simulink model "EHB_MOTOR"  (R2023b)
settings: Solver=FixedStepDiscrete  StartTime=0.0  StopTime=inf  FixedStep=0.0001  RelTol=1e-3  EnableMultiTasking=on
undefined symbols (not defined in the file): CAN_EHB_VCU0x125, CAN_EHB_VCU0x126, CAN_id0x120_Data, Cos_Table, Cos_Table1, EHB_DTC_status, R, Sin_BreakPoint, Sin_BreakPoint1, Sin_Table, Sin_Table1, T
libraries: simulink x30
(part 6 of 9)

== system EHB_MOTOR/EPB_CTRL/EPB_Diag/EPBOverheatDiag/Subsystem1 ==
  note: 控制器温度超过限定值
  In1 : Inport
  function : TriggerPort  TriggerType=function-call  VariantControl=Variant
  Constant : Constant  Value=0  OutDataTypeStr=uint8
  Data Store Memory1 : DataStoreMemory  DataStoreName=EPBTempOverride_C  ReadBeforeWriteMsg=warning  WriteAfterWriteMsg=warning  WriteAfterReadMsg=warning  ShowAdditionalParam=off  OutDataTypeStr=uint16
  Data Store Memory5 : DataStoreMemory  DataStoreName=EPBTempMAX_C  ReadBeforeWriteMsg=warning  WriteAfterWriteMsg=warning  WriteAfterReadMsg=warning  ShowAdditionalParam=off  OutDataTypeStr=uint16
  Data Store Read : DataStoreRead  DataStoreName=EPBTempOverride_C  DataStoreElements=EPBTempOverride_C  IndexOptions=Index vector (dialog)  Indices=1  OutputSizes=1
  Data Store Read2 : DataStoreRead  DataStoreName=EPBTempMAX_C  DataStoreElements=EPBTempMAX_C  IndexOptions=Index vector (dialog)  Indices=1  OutputSizes=1
  ErrorSignalCount : Stateflow chart  TreatAsAtomicUnit=on
  Relational Operator1 : RelationalOperator  Operator=>  OutDataTypeStr=boolean  RndMeth=Simplest  InputSameDT=off
  Out1 : Outport  VectorParamsAs1DForOutWhenUnconnected=off
  wires:
  ErrorSignalCount/1(EPBTempOverride) -> Out1/1
  Relational Operator1/1 -> ErrorSignalCount/1(EPBTemp)
  Data Store Read/1 -> ErrorSignalCount/2(EPBTempOverride_C)
  Constant/1 -> ErrorSignalCount/3(Recover)
  In1/1 -> Relational Operator1/1
  Data Store Read2/1 -> Relational Operator1/2

== system EHB_MOTOR/EPB_CTRL/EPB_Diag/EPB_vBATDiag/Subsystem ==
  note: 电源电压过低
  note: 16V
  note: 10V
  note: 电源电压过高
  In1 : Inport
  function : TriggerPort  TriggerType=function-call  VariantControl=Variant
  Constant : Constant  Value=0  OutDataTypeStr=uint8
  Constant1 : Constant  Value=0  OutDataTypeStr=uint8
  Data Store Memory1 : DataStoreMemory  DataStoreName=EPBVoltage_C  ReadBeforeWriteMsg=warning  WriteAfterWriteMsg=warning  WriteAfterReadMsg=warning  ShowAdditionalParam=off  OutDataTypeStr=uint16
  Data Store Memory4 : DataStoreMemory  DataStoreName=EPBVoltageMIN_C  ReadBeforeWriteMsg=warning  WriteAfterWriteMsg=warning  WriteAfterReadMsg=warning  ShowAdditionalParam=off  OutDataTypeStr=uint16
  Data Store Memory5 : DataStoreMemory  DataStoreName=EPBVoltageMAX_C  ReadBeforeWriteMsg=warning  WriteAfterWriteMsg=warning  WriteAfterReadMsg=warning  ShowAdditionalParam=off  OutDataTypeStr=uint16
  Data Store Read : DataStoreRead  DataStoreName=EPBVoltage_C  DataStoreElements=EPBVoltage_C  IndexOptions=Index vector (dialog)  Indices=1  OutputSizes=1
  Data Store Read1 : DataStoreRead  DataStoreName=EPBVoltageMIN_C  DataStoreElements=EPBVoltageMIN_C  IndexOptions=Index vector (dialog)  Indices=1  OutputSizes=1
  Data Store Read2 : DataStoreRead  DataStoreName=EPBVoltageMAX_C  DataStoreElements=EPBVoltageMAX_C  IndexOptions=Index vector (dialog)  Indices=1  OutputSizes=1
  Data Store Read3 : DataStoreRead  DataStoreName=EPBVoltage_C  DataStoreElements=EPBVoltage_C  IndexOptions=Index vector (dialog)  Indices=1  OutputSizes=1
  ErrorSignalCount : Stateflow chart  TreatAsAtomicUnit=on
  ErrorSignalCount1 : Stateflow chart  TreatAsAtomicUnit=on
  Relational Operator : RelationalOperator  Operator=<  OutDataTypeStr=boolean  RndMeth=Simplest  InputSameDT=off
  Relational Operator1 : RelationalOperator  Operator=>  OutDataTypeStr=boolean  RndMeth=Simplest  InputSameDT=off
  Out1 : Outport  VectorParamsAs1DForOutWhenUnconnected=off
  Out2 : Outport  Port=2  VectorParamsAs1DForOutWhenUnconnected=off
  wires:
  ErrorSignalCount/1(EPBVoltageMAX) -> Out2/1
  Relational Operator1/1 -> ErrorSignalCount/1(EPBVoltage)
  Data Store Read3/1 -> ErrorSignalCount/2(EPBVoltageMAX_C)
  Constant1/1 -> ErrorSignalCount/3(Recover)
  Constant/1 -> ErrorSignalCount1/3(Recover)
  Data Store Read/1 -> ErrorSignalCount1/2(EPBVoltageMIN_C)
  Relational Operator/1 -> ErrorSignalCount1/1(EPBVoltage)
  ErrorSignalCount1/1(EPBVoltageMIN) -> Out1/1
  Data Store Read2/1 -> Relational Operator1/2
  In1/1 -> Relational Operator/1, Relational Operator1/1
  Data Store Read1/1 -> Relational Operator/2

== system EHB_MOTOR/EPB_CTRL/Subsystem1/EPB_interface/12vADC2VOLT ==
  EPB_vBAT_AD : Inport
  Filter : Subsystem  Commented=on
  vMCU2PIN : Subsystem
  EPB_vBAT_filtered : Outport  VectorParamsAs1DForOutWhenUnconnected=off
  wires:
  EPB_vBAT_AD/1 -> vMCU2PIN/1(EPB_vBAT_AD)
  vMCU2PIN/1(EPB_vBAT) -> EPB_vBAT_filtered/1

== system EHB_MOTOR/EPB_CTRL/Subsystem1/EPB_interface/EPB1DC2Cur ==
  EPB1_Current_AD : Inport
  Data Store Memory : DataStoreMemory  DataStoreName=EPB1_actCurent  ReadBeforeWriteMsg=warning  WriteAfterWriteMsg=warning  WriteAfterReadMsg=warning  ShowAdditionalParam=off  OutDataTypeStr=double
  Data Store Write : DataStoreWrite  DataStoreName=EPB1_actCurent  DataStoreElements=EPB1_actCurent  IndexOptions=Index vector (dialog)  Indices=1  OutputSizes=1
  Filter : Subsystem  Commented=on
  vMCU2PIN : Subsystem
  EPB1_Current_filtered : Outport  VectorParamsAs1DForOutWhenUnconnected=off
  wires:
  EPB1_Current_AD/1 -> vMCU2PIN/1(EPB1_Current_AD)
  vMCU2PIN/1(EPB1_Current) -> Data Store Write/1, EPB1_Current_filtered/1

== system EHB_MOTOR/EPB_CTRL/Subsystem1/EPB_interface/EPB2DC2Cur ==
  EPB2_Current_AD : Inport
  Data Store Memory : DataStoreMemory  DataStoreName=EPB2_actCurent  ReadBeforeWriteMsg=warning  WriteAfterWriteMsg=warning  WriteAfterReadMsg=warning  ShowAdditionalParam=off  OutDataTypeStr=double
  Data Store Write : DataStoreWrite  DataStoreName=EPB2_actCurent  DataStoreElements=EPB2_actCurent  IndexOptions=Index vector (dialog)  Indices=1  OutputSizes=1
  Filter : Subsystem  Commented=on
  vMCU2PIN : Subsystem
  EPB2_Current_filtered : Outport  VectorParamsAs1DForOutWhenUnconnected=off
  wires:
  EPB2_Current_AD/1 -> vMCU2PIN/1(EPB2_Current_AD)
  vMCU2PIN/1(EPB2_Current) -> EPB2_Current_filtered/1, Data Store Write/1

== system EHB_MOTOR/EPB_CTRL/Subsystem1/EPB_interface/EPB_7181PreDriver1 ==
  EPB_7181PreDriver1_AD : Inport
  Filter : Subsystem  Commented=on
  vMCU2PIN : Subsystem
  EPB_7181PreDriver1_filtered : Outport  VectorParamsAs1DForOutWhenUnconnected=off
  wires:
  vMCU2PIN/1(EPB_7181PreDriver1) -> EPB_7181PreDriver1_filtered/1
  EPB_7181PreDriver1_AD/1 -> vMCU2PIN/1(EPB_7181PreDriver1_AD)

== system EHB_MOTOR/EPB_CTRL/Subsystem1/EPB_interface/EPB_7181PreDriver2 ==
  EPB_7181PreDriver2_AD : Inport
  Filter : Subsystem  Commented=on
  vMCU2PIN : Subsystem
  EPB_7181PreDriver2_filtered : Outport  VectorParamsAs1DForOutWhenUnconnected=off
  wires:
  EPB_7181PreDriver2_AD/1 -> vMCU2PIN/1(EPB_7181PreDriver2_AD)
  vMCU2PIN/1(EPB_7181PreDriver2) -> EPB_7181PreDriver2_filtered/1

== system EHB_MOTOR/EPB_CTRL/Subsystem1/EPB_interface/EPB_APBSwitch1 ==
  EPB_APBSwitch1_AD : Inport
  Filter : Subsystem  Commented=on
  vMCU2PIN : Subsystem
  EPB_APBSwitch1_filtered : Outport  VectorParamsAs1DForOutWhenUnconnected=off
  wires:
  EPB_APBSwitch1_AD/1 -> vMCU2PIN/1(EPB_APBSwitch1_AD)
  vMCU2PIN/1(EPB_APBSwitch1) -> EPB_APBSwitch1_filtered/1

== system EHB_MOTOR/EPB_CTRL/Subsystem1/EPB_interface/EPB_APBSwitch2 ==
  EPB_APBSwitch2_AD : Inport
  Filter : Subsystem  Commented=on
  vMCU2PIN : Subsystem
  EPB_APBSwitch2_filtered : Outport  VectorParamsAs1DForOutWhenUnconnected=off
  wires:
  vMCU2PIN/1(EPB_APBSwitch2) -> EPB_APBSwitch2_filtered/1
  EPB_APBSwitch2_AD/1 -> vMCU2PIN/1(EPB_APBSwitch2_AD)

== system EHB_MOTOR/EPB_CTRL/Subsystem1/EPB_interface/EPB_APBSwitch3 ==
  EPB_APBSwitch3_AD : Inport
  Filter : Subsystem  Commented=on
  vMCU2PIN : Subsystem
  EPB_APBSwitch3_filtered : Outport  VectorParamsAs1DForOutWhenUnconnected=off
  wires:
  EPB_APBSwitch3_AD/1 -> vMCU2PIN/1(EPB_APBSwitch3_AD)
  vMCU2PIN/1(EPB_APBSwitch3) -> EPB_APBSwitch3_filtered/1

== system EHB_MOTOR/EPB_CTRL/Subsystem1/EPB_interface/EPB_APBSwitch4 ==
  EPB_APBSwitch4_AD : Inport
  Filter : Subsystem  Commented=on
  vMCU2PIN : Subsystem
  EPB_APBSwitch4_filtered : Outport  VectorParamsAs1DForOutWhenUnconnected=off
  wires:
  vMCU2PIN/1(EPB_APBSwitch4) -> EPB_APBSwitch4_filtered/1
  EPB_APBSwitch4_AD/1 -> vMCU2PIN/1(EPB_APBSwitch4_AD)

== system EHB_MOTOR/EPB_CTRL/Subsystem1/EPB_interface/tempADC2Temp ==
  EPB1_Temp_AD : Inport
  Filter : Subsystem  Commented=on
  EPB1_Temp : Outport  VectorParamsAs1DForOutWhenUnconnected=off
  wires:
  EPB1_Temp_AD/1 -> EPB1_Temp/1

== system EHB_MOTOR/EPB_CTRL/Subsystem1/EPB_interface/tempADC2Temp1 ==
  EPB2_Temp_AD : Inport
  Filter : Subsystem  Commented=on
  EPB2_Temp : Outport  VectorParamsAs1DForOutWhenUnconnected=off
  wires:
  EPB2_Temp_AD/1 -> EPB2_Temp/1

== system EHB_MOTOR/EHB_MOTOR_PRO/INPUT/AI/EHB_interface/12vADC2VOLT ==
  EHB_vBAT_AD : Inport
  Data Store Memory : DataStoreMemory  DataStoreName=EHB_12vBAT  ReadBeforeWriteMsg=warning  WriteAfterWriteMsg=warning  WriteAfterReadMsg=warning  ShowAdditionalParam=off  OutDataTypeStr=double
  Data Store Write : DataStoreWrite  DataStoreName=EHB_12vBAT  DataStoreElements=EHB_12vBAT  IndexOptions=Index vector (dialog)  Indices=1  OutputSizes=1
  Filter : Subsystem  Commented=on
  vMCU2PIN : Subsystem
  EHB_vBAT_filtered : Outport  VectorParamsAs1DForOutWhenUnconnected=off
  wires:
  EHB_vBAT_AD/1 -> vMCU2PIN/1(EHB_vBAT_AD)
  vMCU2PIN/1(EHB_vBAT) -> Data Store Write/1, EHB_vBAT_filtered/1

== system EHB_MOTOR/EHB_MOTOR_PRO/INPUT/AI/EHB_interface/12vLogic2VOLT ==
  EHB_12vLogic_AD : Inport
  Data Store Memory : DataStoreMemory  DataStoreName=EHB_12vLogic_filtered  ReadBeforeWriteMsg=warning  WriteAfterWriteMsg=warning  WriteAfterReadMsg=warning  ShowAdditionalParam=off  OutDataTypeStr=double
  Data Store Write : DataStoreWrite  DataStoreName=EHB_12vLogic_filtered  DataStoreElements=EHB_12vLogic_filtered  IndexOptions=Index vector (dialog)  Indices=1  OutputSizes=1
  Filter : Subsystem  Commented=on
  vMCU2PIN : Subsystem
  EHB_12vLogic_filtered : Outport  VectorParamsAs1DForOutWhenUnconnected=off
  wires:
  vMCU2PIN/1(EHB_12vLogic) -> Data Store Write/1, EHB_12vLogic_filtered/1
  EHB_12vLogic_AD/1 -> vMCU2PIN/1(EHB_12vLogic_AD)

== system EHB_MOTOR/EHB_MOTOR_PRO/INPUT/AI/EHB_interface/5vADC2VOLT ==
  EHB_5vOUT_AD : Inport
  Data Store Memory : DataStoreMemory  DataStoreName=EHB_5vACT  ReadBeforeWriteMsg=warning  WriteAfterWriteMsg=warning  WriteAfterReadMsg=warning  ShowAdditionalParam=off  OutDataTypeStr=double
  Data Store Write : DataStoreWrite  DataStoreName=EHB_5vACT  DataStoreElements=EHB_5vACT  IndexOptions=Index vector (dialog)  Indices=1  OutputSizes=1
  Filter : Subsystem  Commented=on
  vMCU2PIN : Subsystem
  EHB_5vOUT_filtered : Outport  VectorParamsAs1DForOutWhenUnconnected=off
  wires:
  EHB_5vOUT_AD/1 -> vMCU2PIN/1(EHB_5vOUT_AD)
  vMCU2PIN/1(EHB_5vOUT) -> EHB_5vOUT_filtered/1, Data Store Write/1

== system EHB_MOTOR/EHB_MOTOR_PRO/INPUT/AI/EHB_interface/KL15ADC2VOLT ==
  EHB_vKL15_AD : Inport
  Data Store Memory : DataStoreMemory  DataStoreName=EHB_KL15vBAT  ReadBeforeWriteMsg=warning  WriteAfterWriteMsg=warning  WriteAfterReadMsg=warning  ShowAdditionalParam=off  OutDataTypeStr=double
  Data Store Write : DataStoreWrite  DataStoreName=EHB_KL15vBAT  DataStoreElements=EHB_KL15vBAT  IndexOptions=Index vector (dialog)  Indices=1  OutputSizes=1
  Filter : Subsystem  Commented=on
  vMCU2PIN : Subsystem
  EHB_vKL15_filtered : Outport  VectorParamsAs1DForOutWhenUnconnected=off
  wires:
  vMCU2PIN/1(EHB_vKL15) -> Data Store Write/1, EHB_vKL15_filtered/1
  EHB_vKL15_AD/1 -> vMCU2PIN/1(EHB_vKL15_AD)

== system EHB_MOTOR/EHB_MOTOR_PRO/INPUT/AI/EHB_interface/Reserve ==
  EHB_Reserve_AD : Inport
  Filter : Subsystem  Commented=on
  vMCU2PIN : Subsystem
  EHB_Reserve_filtered : Outport  VectorParamsAs1DForOutWhenUnconnected=off
  wires:
  vMCU2PIN/1(EHB_Reserve) -> EHB_Reserve_filtered/1
  EHB_Reserve_AD/1 -> vMCU2PIN/1(EHB_Reserve_AD)

== system EHB_MOTOR/EHB_MOTOR_PRO/INPUT/AI/EHB_interface/UADC2Cur ==
  EHB_Ucurrent_AD : Inport
  Data Store Memory : DataStoreMemory  DataStoreName=EHB_iU_filtered  ReadBeforeWriteMsg=warning  WriteAfterWriteMsg=warning  WriteAfterReadMsg=warning  ShowAdditionalParam=off  OutDataTypeStr=single
  Data Store Write : DataStoreWrite  DataStoreName=EHB_iU_filtered  DataStoreElements=EHB_iU_filtered  IndexOptions=Index vector (dialog)  Indices=1  OutputSizes=1
  Filter : Subsystem  Commented=on
  vMCU2PIN : Subsystem
  EHB_iU_filtered : Outport  VectorParamsAs1DForOutWhenUnconnected=off
  wires:
  vMCU2PIN/1(EHB_iU) -> Data Store Write/1, EHB_iU_filtered/1
  EHB_Ucurrent_AD/1 -> vMCU2PIN/1(EHB_Ucurrent_AD)

== system EHB_MOTOR/EHB_MOTOR_PRO/INPUT/AI/EHB_interface/VADC2Cur ==
  EHB_Vcurrent_AD : Inport
  Data Store Memory : DataStoreMemory  DataStoreName=EHB_iV_filtered  ReadBeforeWriteMsg=warning  WriteAfterWriteMsg=warning  WriteAfterReadMsg=warning  ShowAdditionalParam=off  OutDataTypeStr=single
  Data Store Write : DataStoreWrite  DataStoreName=EHB_iV_filtered  DataStoreElements=EHB_iV_filtered  IndexOptions=Index vector (dialog)  Indices=1  OutputSizes=1
  Filter : Subsystem  Commented=on
  vMCU2PIN : Subsystem
  EHB_iV_filtered : Outport  VectorParamsAs1DForOutWhenUnconnected=off
  wires:
  EHB_Vcurrent_AD/1 -> vMCU2PIN/1(EHB_Vcurrent_AD)
  vMCU2PIN/1(EHB_iV) -> Data Store Write/1, EHB_iV_filtered/1

== system EHB_MOTOR/EHB_MOTOR_PRO/INPUT/AI/EHB_interface/VpreADC2Pressure ==
  EHB_Pressure_S1_AD : Inport
  Data Store Memory : DataStoreMemory  DataStoreName=EHB_pwrPressure_filtered  ReadBeforeWriteMsg=warning  WriteAfterWriteMsg=warning  WriteAfterReadMsg=warning  ShowAdditionalParam=off  OutDataTypeStr=double
  Data Store Write : DataStoreWrite  DataStoreName=EHB_pwrPressure_filtered  DataStoreElements=EHB_pwrPressure_filtered  IndexOptions=Index vector (dialog)  Indices=1  OutputSizes=1
  Filter : Subsystem  Commented=on
  vMCU2PIN : Subsystem
  EHB_pwrPressure_filtered : Outport  VectorParamsAs1DForOutWhenUnconnected=off
  wires:
  EHB_Pressure_S1_AD/1 -> vMCU2PIN/1(EHB_Pressure_S1_AD)
  vMCU2PIN/1(vPrePwr_MCU2PIN) -> Data Store Write/1, EHB_pwrPressure_filtered/1

== system EHB_MOTOR/EHB_MOTOR_PRO/INPUT/AI/EHB_interface/WADC2Cur ==
  EHB_Wcurrent_AD : Inport
  Data Store Memory : DataStoreMemory  DataStoreName=EHB_iW_filtered  ReadBeforeWriteMsg=warning  WriteAfterWriteMsg=warning  WriteAfterReadMsg=warning  ShowAdditionalParam=off  OutDataTypeStr=single
  Data Store Write : DataStoreWrite  DataStoreName=EHB_iW_filtered  DataStoreElements=EHB_iW_filtered  IndexOptions=Index vector (dialog)  Indices=1  OutputSizes=1
  Filter : Subsystem  Commented=on
  vMCU2PIN : Subsystem
  EHB_iW_filtered : Outport  VectorParamsAs1DForOutWhenUnconnected=off
  wires:
  vMCU2PIN/1(EHB_iW) -> Data Store Write/1, EHB_iW_filtered/1
  EHB_Wcurrent_AD/1 -> vMCU2PIN/1(EHB_Wcurrent_AD)

== system EHB_MOTOR/EHB_MOTOR_PRO/INPUT/AI/EHB_interface/WheelADC2VOLT ==
  EHB_vWheel_AD : Inport
  Data Store Memory : DataStoreMemory  DataStoreName=EHB_vWheel_filtered  ReadBeforeWriteMsg=warning  WriteAfterWriteMsg=warning  WriteAfterReadMsg=warning  ShowAdditionalParam=off  OutDataTypeStr=double
  Data Store Write : DataStoreWrite  DataStoreName=EHB_vWheel_filtered  DataStoreElements=EHB_vWheel_filtered  IndexOptions=Index vector (dialog)  Indices=1  OutputSizes=1
  Filter : Subsystem  Commented=on
  vMCU2PIN : Subsystem
  EHB_vWheel_filtered : Outport  VectorParamsAs1DForOutWhenUnconnected=off
  wires:
  EHB_vWheel_AD/1 -> vMCU2PIN/1(EHB_vWheel_AD)
  vMCU2PIN/1(EHB_vWheel) -> Data Store Write/1, EHB_vWheel_filtered/1

== system EHB_MOTOR/EHB_MOTOR_PRO/INPUT/AI/EHB_interface/preADC2Presure ==
  note: 压力线性查表，单位Mpa
  note: 求占5v供电的百分比
  EHB_Presure_AD : Inport
  EHB_5vOUT : Inport  Port=2
  1-D Lookup Table : Lookup_n-D  NumberOfTableDimensions=1  BreakpointsForDimension1=[0,10,50,90]  Table=[0,0,15,30]  InternalRulePriority=Speed  RndMeth=Simplest
  Constant : Constant  Value=5
  Constant1 : Constant  Value=100
  Data Store Memory : DataStoreMemory  DataStoreName=EHB_actPresure  ReadBeforeWriteMsg=warning  WriteAfterWriteMsg=warning  WriteAfterReadMsg=warning  ShowAdditionalParam=off  OutDataTypeStr=double
  Data Store Write : DataStoreWrite  DataStoreName=EHB_actPresure  DataStoreElements=EHB_actPresure  IndexOptions=Index vector (dialog)  Indices=1  OutputSizes=1
  Divide : Product  Inputs=*/
  Filter : Subsystem  Commented=on
  Multiply : Product
  Terminator : Terminator
  vMCU2PIN : Subsystem
  EHB_actPresure_filtered : Outport  VectorParamsAs1DForOutWhenUnconnected=off
  wires:
  EHB_Presure_AD/1 -> vMCU2PIN/1(EHB_Presure_AD)
  vMCU2PIN/1(vPre_MCU2PIN) -> Divide/1
  Divide/1 -> Multiply/1
  Constant1/1 -> Multiply/2
  Multiply/1 -> 1-D Lookup Table/1
  1-D Lookup Table/1 -> Data Store Write/1, EHB_actPresure_filtered/1
  EHB_5vOUT/1 -> Terminator/1
  Constant/1 -> Divide/2

== system EHB_MOTOR/EHB_MOTOR_PRO/INPUT/AI/EHB_interface/tempADC2Temp ==
  note: 查表温度范围
  EHB_Temp_AD : Inport
  EHB_5vOUT : Inport  Port=2
  1-D Lookup Table : Lookup_n-D  NumberOfTableDimensions=1  BreakpointsForDimension1=R  Table=T  InternalRulePriority=Speed  RndMeth=Simplest
  Data Store Memory : DataStoreMemory  DataStoreName=EHB_TEMP  ReadBeforeWriteMsg=warning  WriteAfterWriteMsg=warning  WriteAfterReadMsg=warning  ShowAdditionalParam=off  OutDataTypeStr=double
  Data Store Write : DataStoreWrite  DataStoreName=EHB_TEMP  DataStoreElements=EHB_TEMP  IndexOptions=Index vector (dialog)  Indices=1  OutputSizes=1
  Filter : Subsystem  Commented=on
  Subsystem : Subsystem
  EHB_Temp : Outport  VectorParamsAs1DForOutWhenUnconnected=off
  wires:
  EHB_Temp_AD/1 -> Subsystem/1(EHB_Temp_AD)
  Subsystem/1(MOS_rTemp) -> 1-D Lookup Table/1
  1-D Lookup Table/1 -> EHB_Temp/1, Data Store Write/1
  EHB_5vOUT/1 -> Subsystem/2(EHB_5vOUT)

== system EHB_MOTOR/EHB_MOTOR_PRO/Subsystem/Current_PI/Id_PI/Subsystem ==
  In1 : Inport
  In2 : Inport  Port=2
  Constant : Constant  Value=0  OutDataTypeStr=single
  Constant1 : Constant  Value=0  OutDataTypeStr=single
  Relational Operator : RelationalOperator  Operator===  OutDataTypeStr=boolean  RndMeth=Simplest  InputSameDT=off
  Switch : Switch  Criteria=u2 ~= 0  SaturateOnIntegerOverflow=off  InputSameDT=off
  Out1 : Outport  VectorParamsAs1DForOutWhenUnconnected=off
  wires:
  Constant/1 -> Relational Operator/2
  In1/1 -> Relational Operator/1
  Constant1/1 -> Switch/1
  Relational Operator/1 -> Switch/2
  Switch/1 -> Out1/1
  In2/1 -> Switch/3

== system EHB_MOTOR/EHB_MOTOR_PRO/Subsystem/Current_PI/Id_PI/Subsystem1 ==
  In1 : Inport
  In2 : Inport  Port=2
  Constant : Constant  Value=0  OutDataTypeStr=single
  Constant1 : Constant  Value=0  OutDataTypeStr=single
  Relational Operator : RelationalOperator  Operator===  OutDataTypeStr=boolean  RndMeth=Simplest  InputSameDT=off
  Switch : Switch  Criteria=u2 ~= 0  SaturateOnIntegerOverflow=off  InputSameDT=off
  Out1 : Outport  VectorParamsAs1DForOutWhenUnconnected=off
  wires:
  In2/1 -> Switch/3
  Switch/1 -> Out1/1
  Relational Operator/1 -> Switch/2
  Constant1/1 -> Switch/1
  In1/1 -> Relational Operator/1
  Constant/1 -> Relational Operator/2

== system EHB_MOTOR/EHB_MOTOR_PRO/Subsystem/Current_PI/Id_PI/Subsystem2 ==
  In1 : Inport
  In2 : Inport  Port=2
  Constant : Constant  Value=0  OutDataTypeStr=single
  Constant1 : Constant  Value=0  OutDataTypeStr=single
  Relational Operator : RelationalOperator  Operator===  OutDataTypeStr=boolean  RndMeth=Simplest  InputSameDT=off
  Switch : Switch  Criteria=u2 ~= 0  SaturateOnIntegerOverflow=off  InputSameDT=off
  Out1 : Outport  VectorParamsAs1DForOutWhenUnconnected=off
  wires:
  Constant/1 -> Relational Operator/2
  In1/1 -> Relational Operator/1
  Constant1/1 -> Switch/1
  Relational Operator/1 -> Switch/2
  Switch/1 -> Out1/1
  In2/1 -> Switch/3

== system EHB_MOTOR/EHB_MOTOR_PRO/Subsystem/SVPWM/Calculate_Phase_Voltages/Phase_Voltage_Sectors_1_and_4 ==
  Bus_Alpha_Beta : Inport
  Add : Sum  Inputs=+++
  Add1 : Sum  Inputs=+-+
  Add2 : Sum  Inputs=+--
  Bus Creator1 : BusCreator  Inputs=3
  Bus Selector : BusSelector  OutputSignals=Bus_Voltage,U_alpha,U_beta
  Bus Selector1 : BusSelector  OutputSignals=Bus_Voltage,U_alpha,U_beta
  Bus Selector2 : BusSelector  OutputSignals=Bus_Voltage,U_alpha,U_beta
  Gain : Gain  Gain=2  OutDataTypeStr=Inherit: Same as input
  Gain1 : Gain  Gain=sqrt(3)  OutDataTypeStr=Inherit: Same as input
  Gain2 : Gain  Gain=0.25  OutDataTypeStr=Inherit: Same as input
  Gain3 : Gain  Gain=2  OutDataTypeStr=Inherit: Same as input
  Gain4 : Gain  Gain=sqrt(3)  OutDataTypeStr=Inherit: Same as input
  Gain5 : Gain  Gain=0.25  OutDataTypeStr=Inherit: Same as input
  Gain6 : Gain  Gain=3  OutDataTypeStr=Inherit: Same as input
  Gain7 : Gain  Gain=2  OutDataTypeStr=Inherit: Same as input
  Gain8 : Gain  Gain=sqrt(3)  OutDataTypeStr=Inherit: Same as input
  Gain9 : Gain  Gain=0.25  OutDataTypeStr=Inherit: Same as input
  UVW_Sector_1_and_4 : Outport  VectorParamsAs1DForOutWhenUnconnected=off
  wires:
  Gain2/1 -> Bus Creator1/1  "U_duty"
  Bus Selector/1 -> Gain/1  "<Bus_Voltage>"
  Bus Selector/3 -> Add/3  "<U_beta>"
  Gain/1 -> Add/1
  Add/1 -> Gain2/1
  Gain1/1 -> Add/2
  Bus Selector/2 -> Gain1/1  "<U_alpha>"
  Gain6/1 -> Add1/3
  Gain4/1 -> Add1/2
  Bus Selector1/3 -> Gain6/1  "<U_beta>"
  Gain3/1 -> Add1/1
  Add1/1 -> Gain5/1
  Bus Selector1/1 -> Gain3/1  "<Bus_Voltage>"
  Gain5/1 -> Bus Creator1/2  "V_Duty"
  Bus Selector1/2 -> Gain4/1  "<U_alpha>"
  Add2/1 -> Gain9/1
  Gain8/1 -> Add2/2
  Gain7/1 -> Add2/1
  Bus_Alpha_Beta/1 -> Bus Selector2/1, Bus Selector/1, Bus Selector1/1
  Bus Selector2/2 -> Gain8/1  "<U_alpha>"
  Bus Selector2/3 -> Add2/3  "<U_beta>"
  Gain9/1 -> Bus Creator1/3  "W_Duty"
  Bus Selector2/1 -> Gain7/1  "<Bus_Voltage>"
  Bus Creator1/1 -> UVW_Sector_1_and_4/1

== system EHB_MOTOR/EHB_MOTOR_PRO/Subsystem/SVPWM/Calculate_Phase_Voltages/U_Sectors_2_and_5 ==
  Bus_Alpha : Inport
  Add : Sum
  Add1 : Sum  OutDataTypeStr=single
  Add2 : Sum  Inputs=+-
  Bus Creator2 : BusCreator  Inputs=3
  Bus Selector : BusSelector  OutputSignals=Bus_Voltage,U_alpha
  Bus Selector1 : BusSelector  OutputSignals=Bus_Voltage,U_beta
  Bus Selector2 : BusSelector  OutputSignals=Bus_Voltage,U_beta
  Gain1 : Gain  Gain=sqrt(3)  OutDataTypeStr=Inherit: Same as input
  Gain2 : Gain  Gain=0.5  OutDataTypeStr=Inherit: Same as input
  Gain3 : Gain  Gain=0.5  OutDataTypeStr=Inherit: Same as input
  Gain4 : Gain  Gain=0.5  OutDataTypeStr=Inherit: Same as input
  UVW_Sector_2_and_5 : Outport  VectorParamsAs1DForOutWhenUnconnected=off
  wires:
  Bus Selector/2 -> Gain1/1  "<U_alpha>"
  Gain1/1 -> Add/2
  Add/1 -> Gain2/1
  Bus Selector/1 -> Add/1  "<Bus_Voltage>"
  Bus Selector1/1 -> Add1/1  "<Bus_Voltage>"
  Bus_Alpha/1 -> Bus Selector2/1, Bus Selector1/1, Bus Selector/1  "Bus_Beta"
  Bus Selector1/2 -> Add1/2  "<U_beta>"
  Add1/1 -> Gain3/1
  Add2/1 -> Gain4/1
  Bus Selector2/1 -> Add2/1  "<Bus_Voltage>"
  Gain4/1 -> Bus Creator2/3
  Bus Selector2/2 -> Add2/2  "<U_beta>"
  Gain2/1 -> Bus Creator2/1
  Gain3/1 -> Bus Creator2/2
  Bus Creator2/1 -> UVW_Sector_2_and_5/1

== system EHB_MOTOR/EHB_MOTOR_PRO/Subsystem/SVPWM/Calculate_Phase_Voltages/U_Sectors_3_and_6 ==
  Bus_Beta : Inport
  Add : Sum  Inputs=++-  OutDataTypeStr=single
  Add1 : Sum  Inputs=+-+  OutDataTypeStr=single
  Add2 : Sum  Inputs=+--  OutDataTypeStr=single
  Bus Creator3 : BusCreator  Inputs=3
  Bus Selector : BusSelector  OutputSignals=Bus_Voltage,U_alpha,U_beta
  Bus Selector1 : BusSelector  OutputSignals=Bus_Voltage,U_alpha,U_beta
  Bus Selector2 : BusSelector  OutputSignals=Bus_Voltage,U_alpha,U_beta
  Gain : Gain  Gain=2  OutDataTypeStr=Inherit: Same as input
  Gain1 : Gain  Gain=sqrt(3)  OutDataTypeStr=Inherit: Same as input
  Gain10 : Gain  Gain=3  OutDataTypeStr=Inherit: Same as input
  Gain2 : Gain  Gain=0.25  OutDataTypeStr=Inherit: Same as input
  Gain4 : Gain  Gain=2  OutDataTypeStr=Inherit: Same as input
  Gain5 : Gain  Gain=sqrt(3)  OutDataTypeStr=Inherit: Same as input
  Gain6 : Gain  Gain=0.25  OutDataTypeStr=Inherit: Same as input
  Gain7 : Gain  Gain=2  OutDataTypeStr=Inherit: Same as input
  Gain8 : Gain  Gain=sqrt(3)  OutDataTypeStr=Inherit: Same as input
  Gain9 : Gain  Gain=0.25  OutDataTypeStr=Inherit: Same as input
  UVW_Sector_3_and_6 : Outport  OutDataTypeStr=single  VectorParamsAs1DForOutWhenUnconnected=off
  wires:
  Bus Selector/1 -> Gain/1  "<Bus_Voltage>"
  Add/1 -> Gain2/1
  Bus Selector/3 -> Add/3  "<U_beta>"
  Gain/1 -> Add/1
  Gain1/1 -> Add/2
  Bus Selector/2 -> Gain1/1  "<U_alpha>"
  Bus Selector1/1 -> Gain4/1  "<Bus_Voltage>"
  Bus Selector1/2 -> Gain5/1  "<U_alpha>"
  Gain5/1 -> Add1/2
  Gain4/1 -> Add1/1
  Bus_Beta/1 -> Bus Selector2/1, Bus Selector1/1, Bus Selector/1  "Bus_Beta"
  Bus Selector1/3 -> Add1/3  "<U_beta>"
  Add1/1 -> Gain6/1
  Bus Selector2/2 -> Gain8/1  "<U_alpha>"
  Gain7/1 -> Add2/1
  Gain10/1 -> Add2/3
  Gain8/1 -> Add2/2
  Add2/1 -> Gain9/1
  Bus Selector2/3 -> Gain10/1  "<U_beta>"
  Bus Selector2/1 -> Gain7/1  "<Bus_Voltage>"
  Gain2/1 -> Bus Creator3/1
  Gain6/1 -> Bus Creator3/2
  Gain9/1 -> Bus Creator3/3
  Bus Creator3/1 -> UVW_Sector_3_and_6/1

== system EHB_MOTOR/EPB_CTRL/Subsystem1/EPB_interface/12vADC2VOLT/Filter ==
  EPB_vBAT : Inport
  Chart : Stateflow chart  TreatAsAtomicUnit=on
  Data Store Memory : DataStoreMemory  DataStoreName=EPB_vBATfilter_C  ReadBeforeWriteMsg=warning  WriteAfterWriteMsg=warning  WriteAfterReadMsg=warning  ShowAdditionalParam=off  OutDataTypeStr=uint8
  Data Store Read : DataStoreRead  DataStoreName=EPB_vBATfilter_C  DataStoreElements=EPB_vBATfilter_C  IndexOptions=Index vector (dialog)  Indices=1  OutputSizes=1
  EPB_vBAT_filtered : Outport  VectorParamsAs1DForOutWhenUnconnected=off
  wires:
  EPB_vBAT/1 -> Chart/1(input)
  Chart/1(output) -> EPB_vBAT_filtered/1
  Data Store Read/1 -> Chart/2(Filter_C)

== system EHB_MOTOR/EPB_CTRL/Subsystem1/EPB_interface/12vADC2VOLT/vMCU2PIN ==
  note: 运放比例系数
  note: 计算进入主芯片的电压值
  EPB_vBAT_AD : Inport
  Constant : Constant  Value=10/40
  Constant1 : Constant  Value=5/4095
  Divide : Product  Inputs=*/
  Multiply : Product
  EPB_vBAT : Outport  VectorParamsAs1DForOutWhenUnconnected=off
  wires:
  Constant/1 -> Divide/2
  Constant1/1 -> Multiply/2
  Multiply/1 -> Divide/1
  Divide/1 -> EPB_vBAT/1
  EPB_vBAT_AD/1 -> Multiply/1

== system EHB_MOTOR/EPB_CTRL/Subsystem1/EPB_interface/EPB1DC2Cur/Filter ==
  EPB1_Current : Inport
  Chart : Stateflow chart  TreatAsAtomicUnit=on
  Data Store Memory : DataStoreMemory  DataStoreName=EPB1_Current_filter_C  ReadBeforeWriteMsg=warning  WriteAfterWriteMsg=warning  WriteAfterReadMsg=warning  ShowAdditionalParam=off  OutDataTypeStr=uint8
  Data Store Read : DataStoreRead  DataStoreName=EPB1_Current_filter_C  DataStoreElements=EPB1_Current_filter_C  IndexOptions=Index vector (dialog)  Indices=1  OutputSizes=1
  EPB1_Current_filtered : Outport  VectorParamsAs1DForOutWhenUnconnected=off
  wires:
  Data Store Read/1 -> Chart/2(Filter_C)
  Chart/1(output) -> EPB1_Current_filtered/1
  EPB1_Current/1 -> Chart/1(input)

== system EHB_MOTOR/EPB_CTRL/Subsystem1/EPB_interface/EPB1DC2Cur/vMCU2PIN ==
  note: 零位1000
  note: 单位A
  note: 计算进入主芯片的电压值
  note: 采样电阻及运放系数
  EPB1_Current_AD : Inport
  Add : Sum  Inputs=+-
  Constant1 : Constant  Value=5/4095
  Constant2 : Constant  Value=1000
  Constant3 : Constant  Value=0.04
  Divide1 : Product  Inputs=*/
  Multiply : Product
  EPB1_Current : Outport  VectorParamsAs1DForOutWhenUnconnected=off
  wires:
  EPB1_Current_AD/1 -> Add/1
  Multiply/1 -> Divide1/1
  Constant1/1 -> Multiply/2
  Constant2/1 -> Add/2
  Add/1 -> Multiply/1
  Divide1/1 -> EPB1_Current/1
  Constant3/1 -> Divide1/2

== system EHB_MOTOR/EPB_CTRL/Subsystem1/EPB_interface/EPB2DC2Cur/Filter ==
  EPB2_Current : Inport
  Chart : Stateflow chart  TreatAsAtomicUnit=on
  Data Store Memory : DataStoreMemory  DataStoreName=EPB2_Current_filter_C  ReadBeforeWriteMsg=warning  WriteAfterWriteMsg=warning  WriteAfterReadMsg=warning  ShowAdditionalParam=off  OutDataTypeStr=uint8
  Data Store Read : DataStoreRead  DataStoreName=EPB2_Current_filter_C  DataStoreElements=EPB2_Current_filter_C  IndexOptions=Index vector (dialog)  Indices=1  OutputSizes=1
  EPB2_Current_filtered : Outport  VectorParamsAs1DForOutWhenUnconnected=off
  wires:
  EPB2_Current/1 -> Chart/1(input)
  Chart/1(output) -> EPB2_Current_filtered/1
  Data Store Read/1 -> Chart/2(Filter_C)

== system EHB_MOTOR/EPB_CTRL/Subsystem1/EPB_interface/EPB2DC2Cur/vMCU2PIN ==
  note: 零位993
  note: 单位A
  note: 计算进入主芯片的电压值
  note: 采样电阻及运放系数
  EPB2_Current_AD : Inport
  Add : Sum  Inputs=+-
  Constant1 : Constant  Value=5/4095
  Constant2 : Constant  Value=993
  Constant3 : Constant  Value=0.04
  Divide1 : Product  Inputs=*/
  Multiply : Product
  EPB2_Current : Outport  VectorParamsAs1DForOutWhenUnconnected=off
  wires:
  Divide1/1 -> EPB2_Current/1
  Add/1 -> Multiply/1
  Constant2/1 -> Add/2
  Constant1/1 -> Multiply/2
  Multiply/1 -> Divide1/1
  EPB2_Current_AD/1 -> Add/1
  Constant3/1 -> Divide1/2

== system EHB_MOTOR/EPB_CTRL/Subsystem1/EPB_interface/EPB_7181PreDriver1/Filter ==
  EPB_7181PreDriver1 : Inport
  Chart : Stateflow chart  TreatAsAtomicUnit=on
  Data Store Memory : DataStoreMemory  DataStoreName=EPB_7181PreDriver1_C  ReadBeforeWriteMsg=warning  WriteAfterWriteMsg=warning  WriteAfterReadMsg=warning  ShowAdditionalParam=off  OutDataTypeStr=uint8
  Data Store Read : DataStoreRead  DataStoreName=EPB_7181PreDriver1_C  DataStoreElements=EPB_7181PreDriver1_C  IndexOptions=Index vector (dialog)  Indices=1  OutputSizes=1
  EPB_7181PreDriver1_filtered : Outport  VectorParamsAs1DForOutWhenUnconnected=off
  wires:
  Data Store Read/1 -> Chart/2(Filter_C)
  Chart/1(output) -> EPB_7181PreDriver1_filtered/1
  EPB_7181PreDriver1/1 -> Chart/1(input)

== system EHB_MOTOR/EPB_CTRL/Subsystem1/EPB_interface/EPB_7181PreDriver1/vMCU2PIN ==
  note: 计算进入主芯片的电压值
  note: 运放比例系数
  EPB_7181PreDriver1_AD : Inport
  Constant : Constant  Value=10/40
  Constant1 : Constant  Value=5/4095
  Divide : Product  Inputs=*/
  Multiply : Product
  EPB_7181PreDriver1 : Outport  VectorParamsAs1DForOutWhenUnconnected=off
  wires:
  EPB_7181PreDriver1_AD/1 -> Multiply/1
  Divide/1 -> EPB_7181PreDriver1/1
  Multiply/1 -> Divide/1
  Constant1/1 -> Multiply/2
  Constant/1 -> Divide/2

== system EHB_MOTOR/EPB_CTRL/Subsystem1/EPB_interface/EPB_7181PreDriver2/Filter ==
  EPB_7181PreDriver2 : Inport
  Chart : Stateflow chart  TreatAsAtomicUnit=on
  Data Store Memory : DataStoreMemory  DataStoreName=EPB_7181PreDriver2_C  ReadBeforeWriteMsg=warning  WriteAfterWriteMsg=warning  WriteAfterReadMsg=warning  ShowAdditionalParam=off  OutDataTypeStr=uint8
  Data Store Read : DataStoreRead  DataStoreName=EPB_7181PreDriver2_C  DataStoreElements=EPB_7181PreDriver2_C  IndexOptions=Index vector (dialog)  Indices=1  OutputSizes=1
  EPB_7181PreDriver2_filtered : Outport  VectorParamsAs1DForOutWhenUnconnected=off
  wires:
  EPB_7181PreDriver2/1 -> Chart/1(input)
  Chart/1(output) -> EPB_7181PreDriver2_filtered/1
  Data Store Read/1 -> Chart/2(Filter_C)

== system EHB_MOTOR/EPB_CTRL/Subsystem1/EPB_interface/EPB_7181PreDriver2/vMCU2PIN ==
  note: 运放比例系数
  note: 计算进入主芯片的电压值
  EPB_7181PreDriver2_AD : Inport
  Constant : Constant  Value=10/40
  Constant1 : Constant  Value=5/4095
  Divide : Product  Inputs=*/
  Multiply : Product
  EPB_7181PreDriver2 : Outport  VectorParamsAs1DForOutWhenUnconnected=off
  wires:
  Constant/1 -> Divide/2
  Constant1/1 -> Multiply/2
  Multiply/1 -> Divide/1
  Divide/1 -> EPB_7181PreDriver2/1
  EPB_7181PreDriver2_AD/1 -> Multiply/1

== system EHB_MOTOR/EPB_CTRL/Subsystem1/EPB_interface/EPB_APBSwitch1/Filter ==
  EPB_APBSwitch1 : Inport
  Chart : Stateflow chart  TreatAsAtomicUnit=on
  Data Store Memory : DataStoreMemory  DataStoreName=EPB_APBSwitch1_C  ReadBeforeWriteMsg=warning  WriteAfterWriteMsg=warning  WriteAfterReadMsg=warning  ShowAdditionalParam=off  OutDataTypeStr=uint8
  Data Store Read : DataStoreRead  DataStoreName=EPB_APBSwitch1_C  DataStoreElements=EPB_APBSwitch1_C  IndexOptions=Index vector (dialog)  Indices=1  OutputSizes=1
  EPB_APBSwitch1_filtered : Outport  VectorParamsAs1DForOutWhenUnconnected=off
  wires:
  EPB_APBSwitch1/1 -> Chart/1(input)
  Chart/1(output) -> EPB_APBSwitch1_filtered/1
  Data Store Read/1 -> Chart/2(Filter_C)

== system EHB_MOTOR/EPB_CTRL/Subsystem1/EPB_interface/EPB_APBSwitch1/vMCU2PIN ==
  note: 运放比例系数
  note: 计算进入主芯片的电压值
  EPB_APBSwitch1_AD : Inport
  Constant : Constant  Value=10/40
  Constant1 : Constant  Value=5/4095
  Divide : Product  Inputs=*/
  Multiply : Product
  EPB_APBSwitch1 : Outport  VectorParamsAs1DForOutWhenUnconnected=off
  wires:
  Constant/1 -> Divide/2
  Constant1/1 -> Multiply/2
  Multiply/1 -> Divide/1
  Divide/1 -> EPB_APBSwitch1/1
  EPB_APBSwitch1_AD/1 -> Multiply/1

== system EHB_MOTOR/EPB_CTRL/Subsystem1/EPB_interface/EPB_APBSwitch2/Filter ==
  EPB_APBSwitch2 : Inport
  Chart : Stateflow chart  TreatAsAtomicUnit=on
  Data Store Memory : DataStoreMemory  DataStoreName=EPB_APBSwitch2_C  ReadBeforeWriteMsg=warning  WriteAfterWriteMsg=warning  WriteAfterReadMsg=warning  ShowAdditionalParam=off  OutDataTypeStr=uint8
  Data Store Read : DataStoreRead  DataStoreName=EPB_APBSwitch2_C  DataStoreElements=EPB_APBSwitch2_C  IndexOptions=Index vector (dialog)  Indices=1  OutputSizes=1
  EPB_APBSwitch2_filtered : Outport  VectorParamsAs1DForOutWhenUnconnected=off
  wires:
  Data Store Read/1 -> Chart/2(Filter_C)
  Chart/1(output) -> EPB_APBSwitch2_filtered/1
  EPB_APBSwitch2/1 -> Chart/1(input)

== system EHB_MOTOR/EPB_CTRL/Subsystem1/EPB_interface/EPB_APBSwitch2/vMCU2PIN ==
  note: 计算进入主芯片的电压值
  note: 运放比例系数
  EPB_APBSwitch2_AD : Inport
  Constant : Constant  Value=10/40
  Constant1 : Constant  Value=5/4095
  Divide : Product  Inputs=*/
  Multiply : Product
  EPB_APBSwitch2 : Outport  VectorParamsAs1DForOutWhenUnconnected=off
  wires:
  EPB_APBSwitch2_AD/1 -> Multiply/1
  Divide/1 -> EPB_APBSwitch2/1
  Multiply/1 -> Divide/1
  Constant1/1 -> Multiply/2
  Constant/1 -> Divide/2

== system EHB_MOTOR/EPB_CTRL/Subsystem1/EPB_interface/EPB_APBSwitch3/Filter ==
  EPB_APBSwitch3 : Inport
  Chart : Stateflow chart  TreatAsAtomicUnit=on
  Data Store Memory : DataStoreMemory  DataStoreName=EPB_APBSwitch3_C  ReadBeforeWriteMsg=warning  WriteAfterWriteMsg=warning  WriteAfterReadMsg=warning  ShowAdditionalParam=off  OutDataTypeStr=uint8
  Data Store Read : DataStoreRead  DataStoreName=EPB_APBSwitch3_C  DataStoreElements=EPB_APBSwitch3_C  IndexOptions=Index vector (dialog)  Indices=1  OutputSizes=1
  EPB_APBSwitch3_filtered : Outport  VectorParamsAs1DForOutWhenUnconnected=off
  wires:
  EPB_APBSwitch3/1 -> Chart/1(input)
  Chart/1(output) -> EPB_APBSwitch3_filtered/1
  Data Store Read/1 -> Chart/2(Filter_C)

== system EHB_MOTOR/EPB_CTRL/Subsystem1/EPB_interface/EPB_APBSwitch3/vMCU2PIN ==
  note: 运放比例系数
  note: 计算进入主芯片的电压值
  EPB_APBSwitch3_AD : Inport
  Constant : Constant  Value=10/40
  Constant1 : Constant  Value=5/4095
  Divide : Product  Inputs=*/
  Multiply : Product
  EPB_APBSwitch3 : Outport  VectorParamsAs1DForOutWhenUnconnected=off
  wires:
  Constant/1 -> Divide/2
  Constant1/1 -> Multiply/2
  Multiply/1 -> Divide/1
  Divide/1 -> EPB_APBSwitch3/1
  EPB_APBSwitch3_AD/1 -> Multiply/1

== system EHB_MOTOR/EPB_CTRL/Subsystem1/EPB_interface/EPB_APBSwitch4/Filter ==
  EPB_APBSwitch4 : Inport
  Chart : Stateflow chart  TreatAsAtomicUnit=on
  Data Store Memory : DataStoreMemory  DataStoreName=EPB_APBSwitch4_C  ReadBeforeWriteMsg=warning  WriteAfterWriteMsg=warning  WriteAfterReadMsg=warning  ShowAdditionalParam=off  OutDataTypeStr=uint8
  Data Store Read : DataStoreRead  DataStoreName=EPB_APBSwitch4_C  DataStoreElements=EPB_APBSwitch4_C  IndexOptions=Index vector (dialog)  Indices=1  OutputSizes=1
  EPB_APBSwitch4_filtered : Outport  VectorParamsAs1DForOutWhenUnconnected=off
  wires:
  Data Store Read/1 -> Chart/2(Filter_C)
  Chart/1(output) -> EPB_APBSwitch4_filtered/1
  EPB_APBSwitch4/1 -> Chart/1(input)

== system EHB_MOTOR/EPB_CTRL/Subsystem1/EPB_interface/EPB_APBSwitch4/vMCU2PIN ==
  note: 计算进入主芯片的电压值
  note: 运放比例系数
  EPB_APBSwitch4_AD : Inport
  Constant : Constant  Value=10/40
  Constant1 : Constant  Value=5/4095
  Divide : Product  Inputs=*/
  Multiply : Product
  EPB_APBSwitch4 : Outport  VectorParamsAs1DForOutWhenUnconnected=off
  wires:
  EPB_APBSwitch4_AD/1 -> Multiply/1
  Divide/1 -> EPB_APBSwitch4/1
  Multiply/1 -> Divide/1
  Constant1/1 -> Multiply/2
  Constant/1 -> Divide/2

== system EHB_MOTOR/EPB_CTRL/Subsystem1/EPB_interface/tempADC2Temp/Filter ==
  In1 : Inport
  Chart : Stateflow chart  TreatAsAtomicUnit=on
  Out1 : Outport  VectorParamsAs1DForOutWhenUnconnected=off
  wires:
  In1/1 -> Chart/1(input)
  Chart/1(output) -> Out1/1

== system EHB_MOTOR/EPB_CTRL/Subsystem1/EPB_interface/tempADC2Temp1/Filter ==
  In1 : Inport
  Chart : Stateflow chart  TreatAsAtomicUnit=on
  Out1 : Outport  VectorParamsAs1DForOutWhenUnconnected=off
  wires:
  Chart/1(output) -> Out1/1
  In1/1 -> Chart/1(input)

== system EHB_MOTOR/EHB_MOTOR_PRO/INPUT/AI/EHB_interface/12vADC2VOLT/Filter ==
  EHB_vBAT : Inport
  Chart : Stateflow chart  TreatAsAtomicUnit=on
  Data Store Memory : DataStoreMemory  DataStoreName=vBATfilter_C  ReadBeforeWriteMsg=warning  WriteAfterWriteMsg=warning  WriteAfterReadMsg=warning  ShowAdditionalParam=off  OutDataTypeStr=uint8
  Data Store Read : DataStoreRead  DataStoreName=vBATfilter_C  DataStoreElements=vBATfilter_C  IndexOptions=Index vector (dialog)  Indices=1  OutputSizes=1
  EHB_vBAT_filtered : Outport  VectorParamsAs1DForOutWhenUnconnected=off
  wires:
  EHB_vBAT/1 -> Chart/1(input)
  Chart/1(output) -> EHB_vBAT_filtered/1
  Data Store Read/1 -> Chart/2(Filter_C)

== system EHB_MOTOR/EHB_MOTOR_PRO/INPUT/AI/EHB_interface/12vADC2VOLT/vMCU2PIN ==
  note: 运放比例系数
  note: 计算进入主芯片的电压值
  EHB_vBAT_AD : Inport
  Constant : Constant  Value=10/40
  Constant1 : Constant  Value=5/4095
  Divide : Product  Inputs=*/
  Multiply : Product
  EHB_vBAT : Outport  VectorParamsAs1DForOutWhenUnconnected=off
  wires:
  Constant/1 -> Divide/2
  Constant1/1 -> Multiply/2
  Multiply/1 -> Divide/1
  Divide/1 -> EHB_vBAT/1
  EHB_vBAT_AD/1 -> Multiply/1

== system EHB_MOTOR/EHB_MOTOR_PRO/INPUT/AI/EHB_interface/12vLogic2VOLT/Filter ==
  EHB_12vLogic : Inport
  Chart : Stateflow chart  TreatAsAtomicUnit=on
  Data Store Memory : DataStoreMemory  DataStoreName=EHB_12vLogic  ReadBeforeWriteMsg=warning  WriteAfterWriteMsg=warning  WriteAfterReadMsg=warning  ShowAdditionalParam=off  OutDataTypeStr=uint8
  Data Store Read : DataStoreRead  DataStoreName=EHB_12vLogic  DataStoreElements=EHB_12vLogic  IndexOptions=Index vector (dialog)  Indices=1  OutputSizes=1
  EHB_12vLogic_filtered : Outport  VectorParamsAs1DForOutWhenUnconnected=off
  wires:
  Data Store Read/1 -> Chart/2(Filter_C)
  Chart/1(output) -> EHB_12vLogic_filtered/1
  EHB_12vLogic/1 -> Chart/1(input)

== system EHB_MOTOR/EHB_MOTOR_PRO/INPUT/AI/EHB_interface/12vLogic2VOLT/vMCU2PIN ==
  note: 计算进入主芯片的电压值
  note: 运放比例系数
  EHB_12vLogic_AD : Inport
  Constant : Constant  Value=10/40
  Constant1 : Constant  Value=5/4095
  Divide : Product  Inputs=*/
  Multiply : Product
  EHB_12vLogic : Outport  VectorParamsAs1DForOutWhenUnconnected=off
  wires:
  EHB_12vLogic_AD/1 -> Multiply/1
  Divide/1 -> EHB_12vLogic/1
  Multiply/1 -> Divide/1
  Constant1/1 -> Multiply/2
  Constant/1 -> Divide/2

== system EHB_MOTOR/EHB_MOTOR_PRO/INPUT/AI/EHB_interface/5vADC2VOLT/Filter ==
  EHB_5vOUT : Inport
  Chart : Stateflow chart  TreatAsAtomicUnit=on
  Data Store Memory : DataStoreMemory  DataStoreName=v5OUTfilter_C  ReadBeforeWriteMsg=warning  WriteAfterWriteMsg=warning  WriteAfterReadMsg=warning  ShowAdditionalParam=off  OutDataTypeStr=uint8
  Data Store Read : DataStoreRead  DataStoreName=v5OUTfilter_C  DataStoreElements=v5OUTfilter_C  IndexOptions=Index vector (dialog)  Indices=1  OutputSizes=1
  EHB_5vOUT_filtered : Outport  VectorParamsAs1DForOutWhenUnconnected=off
  wires:
  EHB_5vOUT/1 -> Chart/1(input)
  Chart/1(output) -> EHB_5vOUT_filtered/1
  Data Store Read/1 -> Chart/2(Filter_C)

== system EHB_MOTOR/EHB_MOTOR_PRO/INPUT/AI/EHB_interface/5vADC2VOLT/vMCU2PIN ==
  note: 计算进入主芯片的电压值
  note: 运放比例系数
  EHB_5vOUT_AD : Inport
  Constant : Constant  Value=10/40
  Constant1 : Constant  Value=5/4095
  Divide : Product  Inputs=*/
  Multiply : Product
  EHB_5vOUT : Outport  VectorParamsAs1DForOutWhenUnconnected=off
  wires:
  EHB_5vOUT_AD/1 -> Multiply/1
  Divide/1 -> EHB_5vOUT/1
  Multiply/1 -> Divide/1
  Constant1/1 -> Multiply/2
  Constant/1 -> Divide/2

== system EHB_MOTOR/EHB_MOTOR_PRO/INPUT/AI/EHB_interface/KL15ADC2VOLT/Filter ==
  EHB_vKL15 : Inport
  Chart : Stateflow chart  TreatAsAtomicUnit=on
  Data Store Memory : DataStoreMemory  DataStoreName=vKL15filter_C  ReadBeforeWriteMsg=warning  WriteAfterWriteMsg=warning  WriteAfterReadMsg=warning  ShowAdditionalParam=off  OutDataTypeStr=uint8
  Data Store Read : DataStoreRead  DataStoreName=vKL15filter_C  DataStoreElements=vKL15filter_C  IndexOptions=Index vector (dialog)  Indices=1  OutputSizes=1
  EHB_vKL15_filtered : Outport  VectorParamsAs1DForOutWhenUnconnected=off
  wires:
  Data Store Read/1 -> Chart/2(Filter_C)
  Chart/1(output) -> EHB_vKL15_filtered/1
  EHB_vKL15/1 -> Chart/1(input)

== system EHB_MOTOR/EHB_MOTOR_PRO/INPUT/AI/EHB_interface/KL15ADC2VOLT/vMCU2PIN ==
  note: 计算进入主芯片的电压值
  note: 运放比例系数
  EHB_vKL15_AD : Inport
  Constant : Constant  Value=10/40
  Constant1 : Constant  Value=5/4095
  Divide : Product  Inputs=*/
  Multiply : Product
  EHB_vKL15 : Outport  VectorParamsAs1DForOutWhenUnconnected=off
  wires:
  EHB_vKL15_AD/1 -> Multiply/1
  Divide/1 -> EHB_vKL15/1
  Multiply/1 -> Divide/1
  Constant1/1 -> Multiply/2
  Constant/1 -> Divide/2

== system EHB_MOTOR/EHB_MOTOR_PRO/INPUT/AI/EHB_interface/Reserve/Filter ==
  EHB_Reserve : Inport
  Chart : Stateflow chart  TreatAsAtomicUnit=on
  Data Store Memory : DataStoreMemory  DataStoreName=EHB_Reserve  ReadBeforeWriteMsg=warning  WriteAfterWriteMsg=warning  WriteAfterReadMsg=warning  ShowAdditionalParam=off  OutDataTypeStr=uint8
  Data Store Read : DataStoreRead  DataStoreName=EHB_Reserve  DataStoreElements=EHB_Reserve  IndexOptions=Index vector (dialog)  Indices=1  OutputSizes=1
  EHB_Reserve_filtered : Outport  VectorParamsAs1DForOutWhenUnconnected=off
  wires:
  Data Store Read/1 -> Chart/2(Filter_C)
  Chart/1(output) -> EHB_Reserve_filtered/1
  EHB_Reserve/1 -> Chart/1(input)

== system EHB_MOTOR/EHB_MOTOR_PRO/INPUT/AI/EHB_interface/Reserve/vMCU2PIN ==
  note: 计算进入主芯片的电压值
  note: 运放比例系数
  EHB_Reserve_AD : Inport
  Constant : Constant  Value=50/350
  Constant1 : Constant  Value=5/4095
  Divide : Product  Inputs=*/
  Multiply : Product
  EHB_Reserve : Outport  VectorParamsAs1DForOutWhenUnconnected=off
  wires:
  EHB_Reserve_AD/1 -> Multiply/1
  Divide/1 -> EHB_Reserve/1
  Multiply/1 -> Divide/1
  Constant1/1 -> Multiply/2
  Constant/1 -> Divide/2

== system EHB_MOTOR/EHB_MOTOR_PRO/INPUT/AI/EHB_interface/UADC2Cur/Filter ==
  EHB_iU : Inport
  Chart : Stateflow chart  TreatAsAtomicUnit=on
  Data Store Memory : DataStoreMemory  DataStoreName=iUfilter_C  ReadBeforeWriteMsg=warning  WriteAfterWriteMsg=warning  WriteAfterReadMsg=warning  ShowAdditionalParam=off  OutDataTypeStr=uint8
  Data Store Read : DataStoreRead  DataStoreName=iUfilter_C  DataStoreElements=iUfilter_C  IndexOptions=Index vector (dialog)  Indices=1  OutputSizes=1
  EHB_iU_filtered : Outport  VectorParamsAs1DForOutWhenUnconnected=off
  wires:
  Data Store Read/1 -> Chart/2(Filter_C)
  Chart/1(output) -> EHB_iU_filtered/1
  EHB_iU/1 -> Chart/1(input)

== system EHB_MOTOR/EHB_MOTOR_PRO/INPUT/AI/EHB_interface/UADC2Cur/vMCU2PIN ==
  EHB_Ucurrent_AD : Inport
  Add : Sum  Inputs=+-  OutDataTypeStr=int16
  Data Store Read : DataStoreRead  DataStoreName=Uzero_adc  DataStoreElements=Uzero_adc  IndexOptions=Index vector (dialog)  Indices=1  OutputSizes=1
  U_Vot_Cur_coeff : Gain  Gain=0.0814  OutDataTypeStr=single
  EHB_iU : Outport  VectorParamsAs1DForOutWhenUnconnected=off
  wires:
  EHB_Ucurrent_AD/1 -> Add/1
  U_Vot_Cur_coeff/1 -> EHB_iU/1
  Data Store Read/1 -> Add/2
  Add/1 -> U_Vot_Cur_coeff/1

== system EHB_MOTOR/EHB_MOTOR_PRO/INPUT/AI/EHB_interface/VADC2Cur/Filter ==
  EHB_iV : Inport
  Chart : Stateflow chart  TreatAsAtomicUnit=on
  Data Store Memory : DataStoreMemory  DataStoreName=iVfilter_C  ReadBeforeWriteMsg=warning  WriteAfterWriteMsg=warning  WriteAfterReadMsg=warning  ShowAdditionalParam=off  OutDataTypeStr=uint8
  Data Store Read : DataStoreRead  DataStoreName=iVfilter_C  DataStoreElements=iVfilter_C  IndexOptions=Index vector (dialog)  Indices=1  OutputSizes=1
  EHB_iV_filtered : Outport  VectorParamsAs1DForOutWhenUnconnected=off
  wires:
  EHB_iV/1 -> Chart/1(input)
  Chart/1(output) -> EHB_iV_filtered/1
  Data Store Read/1 -> Chart/2(Filter_C)

== system EHB_MOTOR/EHB_MOTOR_PRO/INPUT/AI/EHB_interface/VADC2Cur/vMCU2PIN ==
  EHB_Vcurrent_AD : Inport
  Add : Sum  Inputs=+-  OutDataTypeStr=int16
  Data Store Read : DataStoreRead  DataStoreName=Vzero_adc  DataStoreElements=Vzero_adc  IndexOptions=Index vector (dialog)  Indices=1  OutputSizes=1
  U_Vot_Cur_coeff : Gain  Gain=0.0814  OutDataTypeStr=single
  EHB_iV : Outport  VectorParamsAs1DForOutWhenUnconnected=off
  wires:
  U_Vot_Cur_coeff/1 -> EHB_iV/1
  EHB_Vcurrent_AD/1 -> Add/1
  Data Store Read/1 -> Add/2
  Add/1 -> U_Vot_Cur_coeff/1

== system EHB_MOTOR/EHB_MOTOR_PRO/INPUT/AI/EHB_interface/VpreADC2Pressure/Filter ==
  EHB_actPressure : Inport
  Chart : Stateflow chart  TreatAsAtomicUnit=on
  Data Store Memory : DataStoreMemory  DataStoreName=Prefilter_C  ReadBeforeWriteMsg=warning  WriteAfterWriteMsg=warning  WriteAfterReadMsg=warning  ShowAdditionalParam=off  OutDataTypeStr=uint8
  Data Store Read : DataStoreRead  DataStoreName=Prefilter_C  DataStoreElements=Prefilter_C  IndexOptions=Index vector (dialog)  Indices=1  OutputSizes=1
  EHB_actPressure_filtered : Outport  VectorParamsAs1DForOutWhenUnconnected=off
  wires:
  EHB_actPressure/1 -> Chart/1(input)
  Chart/1(output) -> EHB_actPressure_filtered/1
  Data Store Read/1 -> Chart/2(Filter_C)

== system EHB_MOTOR/EHB_MOTOR_PRO/INPUT/AI/EHB_interface/VpreADC2Pressure/vMCU2PIN ==
  note: 运放比例系数
  note: 计算进入主芯片的电压值
  EHB_Pressure_S1_AD : Inport
  Constant : Constant  Value=10/20
  Constant1 : Constant  Value=5/4095
  Divide : Product  Inputs=*/
  Multiply : Product
  vPrePwr_MCU2PIN : Outport  VectorParamsAs1DForOutWhenUnconnected=off
  wires:
  Constant/1 -> Divide/2
  Constant1/1 -> Multiply/2
  Multiply/1 -> Divide/1
  Divide/1 -> vPrePwr_MCU2PIN/1
  EHB_Pressure_S1_AD/1 -> Multiply/1

== system EHB_MOTOR/EHB_MOTOR_PRO/INPUT/AI/EHB_interface/WADC2Cur/Filter ==
  EHB_iW : Inport
  Chart : Stateflow chart  TreatAsAtomicUnit=on
  Data Store Memory : DataStoreMemory  DataStoreName=iWfilter_C  ReadBeforeWriteMsg=warning  WriteAfterWriteMsg=warning  WriteAfterReadMsg=warning  ShowAdditionalParam=off  OutDataTypeStr=uint8
  Data Store Read : DataStoreRead  DataStoreName=iWfilter_C  DataStoreElements=iWfilter_C  IndexOptions=Index vector (dialog)  Indices=1  OutputSizes=1
  EHB_iW_filtered : Outport  VectorParamsAs1DForOutWhenUnconnected=off
  wires:
  Data Store Read/1 -> Chart/2(Filter_C)
  Chart/1(output) -> EHB_iW_filtered/1
  EHB_iW/1 -> Chart/1(input)

== system EHB_MOTOR/EHB_MOTOR_PRO/INPUT/AI/EHB_interface/WADC2Cur/vMCU2PIN ==
  EHB_Wcurrent_AD : Inport
  Add : Sum  Inputs=+-  OutDataTypeStr=int16
  Data Store Read : DataStoreRead  DataStoreName=Wzero_adc  DataStoreElements=Wzero_adc  IndexOptions=Index vector (dialog)  Indices=1  OutputSizes=1
  U_Vot_Cur_coeff : Gain  Gain=0.0814  OutDataTypeStr=single
  EHB_iW : Outport  VectorParamsAs1DForOutWhenUnconnected=off
  wires:
  U_Vot_Cur_coeff/1 -> EHB_iW/1
  EHB_Wcurrent_AD/1 -> Add/1
  Data Store Read/1 -> Add/2
  Add/1 -> U_Vot_Cur_coeff/1

== system EHB_MOTOR/EHB_MOTOR_PRO/INPUT/AI/EHB_interface/WheelADC2VOLT/Filter ==
  EHB_vWheel : Inport
  Chart : Stateflow chart  TreatAsAtomicUnit=on
  Data Store Memory : DataStoreMemory  DataStoreName=vWheelfilter_C  ReadBeforeWriteMsg=warning  WriteAfterWriteMsg=warning  WriteAfterReadMsg=warning  ShowAdditionalParam=off  OutDataTypeStr=uint8
  Data Store Read : DataStoreRead  DataStoreName=vWheelfilter_C  DataStoreElements=vWheelfilter_C  IndexOptions=Index vector (dialog)  Indices=1  OutputSizes=1
  EHB_vWheel_filtered : Outport  VectorParamsAs1DForOutWhenUnconnected=off
  wires:
  EHB_vWheel/1 -> Chart/1(input)
  Chart/1(output) -> EHB_vWheel_filtered/1
  Data Store Read/1 -> Chart/2(Filter_C)

== system EHB_MOTOR/EHB_MOTOR_PRO/INPUT/AI/EHB_interface/WheelADC2VOLT/vMCU2PIN ==
  note: 运放比例系数
  note: 计算进入主芯片的电压值
  EHB_vWheel_AD : Inport
  Constant : Constant
  Constant1 : Constant  Value=5/4095
  Divide : Product  Inputs=*/
  Multiply : Product
  EHB_vWheel : Outport  VectorParamsAs1DForOutWhenUnconnected=off
  wires:
  Constant/1 -> Divide/2
  Constant1/1 -> Multiply/2
  Multiply/1 -> Divide/1
  Divide/1 -> EHB_vWheel/1
  EHB_vWheel_AD/1 -> Multiply/1

== system EHB_MOTOR/EHB_MOTOR_PRO/INPUT/AI/EHB_interface/preADC2Presure/Filter ==
  EHB_actPresure : Inport
  Chart : Stateflow chart  TreatAsAtomicUnit=on
  Data Store Memory : DataStoreMemory  DataStoreName=Prefilter_C  ReadBeforeWriteMsg=warning  WriteAfterWriteMsg=warning  WriteAfterReadMsg=warning  ShowAdditionalParam=off  OutDataTypeStr=uint8
  Data Store Read : DataStoreRead  DataStoreName=Prefilter_C  DataStoreElements=Prefilter_C  IndexOptions=Index vector (dialog)  Indices=1  OutputSizes=1
  EHB_actPresure_filtered : Outport  VectorParamsAs1DForOutWhenUnconnected=off
  wires:
  EHB_actPresure/1 -> Chart/1(input)
  Chart/1(output) -> EHB_actPresure_filtered/1
  Data Store Read/1 -> Chart/2(Filter_C)
